simulink model "Qtank"  (R2016b)
settings: Solver=ode45  StartTime=0.0  StopTime=200.0  FixedStep=0.1  RelTol=1e-3
values from neighbouring files (symbols this model uses):
  a1 = 0.071    [datos.m]
  A1 = 28    [datos.m]
  A2 = 32    [datos.m]
  a2 = 0.057    [datos.m]
  A3 = 28    [datos.m]
  a3 = 0.071    [datos.m]
  A4 = 32    [datos.m]
  a4 = 0.057    [datos.m]
  g = 981    [datos.m]
  h1_0 = 40    [datos.m]
  h2_0 = 40    [datos.m]
  h3_0 = 40    [datos.m]
  h4_0 = 40    [datos.m]
  k1 = 3.33    [datos.m]
  k2 = 3.33    [datos.m]
  y1 = 0.7    [datos.m]
  y2 = 0.6    [datos.m]
libraries: simulink x2
settings Model: Creator=mathiaslambert  LastModifiedBy=mathiaslambert

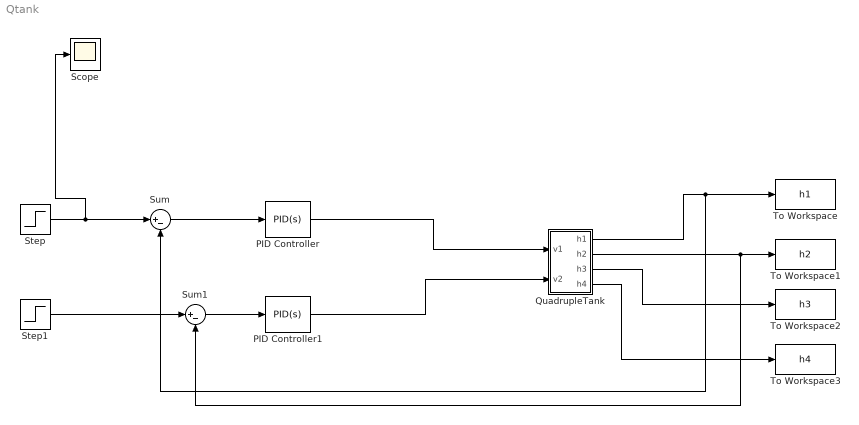
== system Qtank ==
  PID Controller : simulink/Continuous/PID Controller  Controller=PID  TimeDomain=Continuous-time  SampleTime=-1  IntegratorMethod=Forward Euler  FilterMethod=Forward Euler  Form=Parallel  UseFilter=on  ControllerParametersSource=internal  P=0.556896851749042  I=0.0082561633010969  D=-3.05414706908049  N=0.18234120333855  InitialConditionSource=internal  InitialConditionForIntegrator=0  InitialConditionForFilter=0  ExternalReset=none  LimitOutput=on  UpperSaturationLimit=5  LowerSaturationLimit=-5  LinearizeAsGain=on  AntiWindupMode=none  Kb=0.01  TrackingMode=off  Kt=1  PParamMin=[]  PParamMax=[]  IParamMin=[]  IParamMax=[]  DParamMin=[]  DParamMax=[]  NParamMin=[]  NParamMax=[]  KbParamMin=[]  KbParamMax=[]  KtParamMin=[]  KtParamMax=[]  POutMin=[]  POutMax=[]  IOutMin=[]  IOutMax=[]  DOutMin=[]  DOutMax=[]  NOutMin=[]  NOutMax=[]  KbOutMin=[]  KbOutMax=[]  KtOutMin=[]  KtOutMax=[]  IntegratorOutMin=[]  IntegratorOutMax=[]  FilterOutMin=[]  FilterOutMax=[]  SumOutMin=[]  SumOutMax=[]  SumI1OutMin=[]  SumI1OutMax=[]  SumI2OutMin=[]  SumI2OutMax=[]  SumI3OutMin=[]  SumI3OutMax=[]  SumDOutMin=[]  SumDOutMax=[]  SaturationOutMin=[]  SaturationOutMax=[]  IntegratorContinuousStateAttributes=''  IntegratorStateMustResolveToSignalObject=off  IntegratorRTWStateStorageClass=Auto  FilterContinuousStateAttributes=''  FilterStateMustResolveToSignalObject=off  FilterRTWStateStorageClass=Auto  DifferentiatorICPrevScaledInput=0  DifferentiatorOutMin=[]  DifferentiatorOutMax=[]
  PID Controller1 : simulink/Continuous/PID Controller  Controller=PID  TimeDomain=Continuous-time  SampleTime=-1  IntegratorMethod=Forward Euler  FilterMethod=Forward Euler  Form=Parallel  UseFilter=on  ControllerParametersSource=internal  P=1.02825937558598  I=0.0188425600987608  D=-0.134962487418389  N=7.61885317361069  InitialConditionSource=internal  InitialConditionForIntegrator=0  InitialConditionForFilter=0  ExternalReset=none  LimitOutput=on  UpperSaturationLimit=5  LowerSaturationLimit=-5  LinearizeAsGain=on  AntiWindupMode=none  Kb=0.01  TrackingMode=off  Kt=1  PParamMin=[]  PParamMax=[]  IParamMin=[]  IParamMax=[]  DParamMin=[]  DParamMax=[]  NParamMin=[]  NParamMax=[]  KbParamMin=[]  KbParamMax=[]  KtParamMin=[]  KtParamMax=[]  POutMin=[]  POutMax=[]  IOutMin=[]  IOutMax=[]  DOutMin=[]  DOutMax=[]  NOutMin=[]  NOutMax=[]  KbOutMin=[]  KbOutMax=[]  KtOutMin=[]  KtOutMax=[]  IntegratorOutMin=[]  IntegratorOutMax=[]  FilterOutMin=[]  FilterOutMax=[]  SumOutMin=[]  SumOutMax=[]  SumI1OutMin=[]  SumI1OutMax=[]  SumI2OutMin=[]  SumI2OutMax=[]  SumI3OutMin=[]  SumI3OutMax=[]  SumDOutMin=[]  SumDOutMax=[]  SaturationOutMin=[]  SaturationOutMax=[]  IntegratorContinuousStateAttributes=''  IntegratorStateMustResolveToSignalObject=off  IntegratorRTWStateStorageClass=Auto  FilterContinuousStateAttributes=''  FilterStateMustResolveToSignalObject=off  FilterRTWStateStorageClass=Auto  DifferentiatorICPrevScaledInput=0  DifferentiatorOutMin=[]  DifferentiatorOutMax=[]
  QuadrupleTank : Subsystem
  Scope : Scope
  Step : Step  Time=100  Before=40  After=45  SampleTime=0
  Step1 : Step  Time=100  Before=40  After=45  SampleTime=0
  Sum : Sum  Inputs=|+-
  Sum1 : Sum  Inputs=|+-
  To Workspace : ToWorkspace  VariableName=h1  SaveFormat=Timeseries  SampleTime=-1
  To Workspace1 : ToWorkspace  VariableName=h2  SaveFormat=Timeseries  SampleTime=-1
  To Workspace2 : ToWorkspace  VariableName=h3  SaveFormat=Timeseries  SampleTime=-1
  To Workspace3 : ToWorkspace  VariableName=h4  SaveFormat=Timeseries  SampleTime=-1
  wires:
  QuadrupleTank/1(h1) -> Sum/2, To Workspace/1
  QuadrupleTank/2(h2) -> Sum1/2, To Workspace1/1
  QuadrupleTank/3(h3) -> To Workspace2/1
  QuadrupleTank/4(h4) -> To Workspace3/1
  Step1/1 -> Sum1/1
  Step/1 -> Scope/1, Sum/1
  Sum1/1 -> PID Controller1/1
  Sum/1 -> PID Controller/1
  PID Controller/1 -> QuadrupleTank/1(v1)
  PID Controller1/1 -> QuadrupleTank/2(v2)

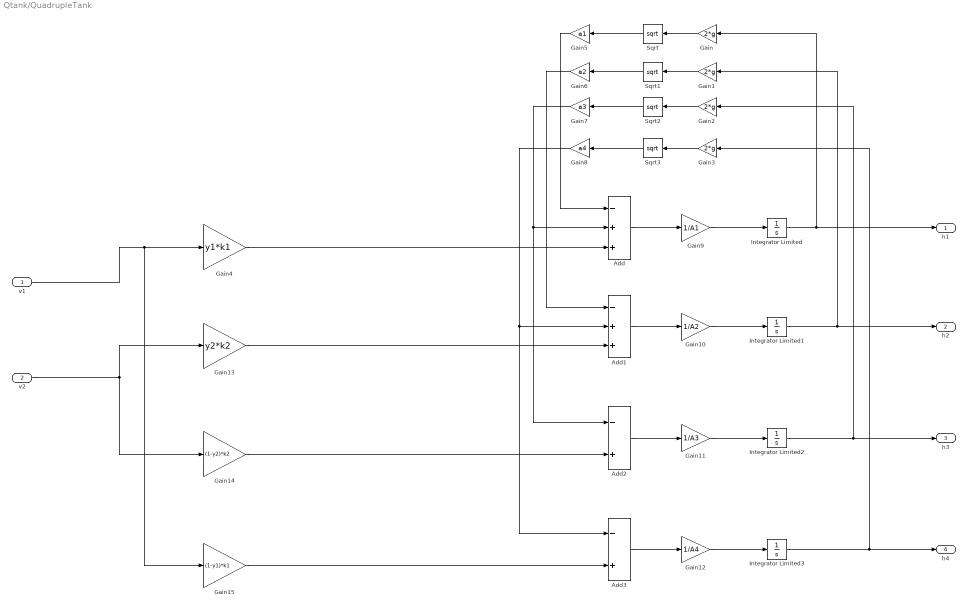
== system Qtank/QuadrupleTank ==
  v1 : Inport
  v2 : Inport  Port=2
  Add : Sum  Inputs=-++
  Add1 : Sum  Inputs=-++
  Add2 : Sum  Inputs=-+
  Add3 : Sum  Inputs=-+
  Gain{,1..3} (4 alike) : Gain  Gain=2*g
  Gain10 : Gain  Gain=1/A2
  Gain11 : Gain  Gain=1/A3
  Gain12 : Gain  Gain=1/A4
  Gain13 : Gain  Gain=y2*k2
  Gain14 : Gain  Gain=(1-y2)*k2
  Gain15 : Gain  Gain=(1-y1)*k1
  Gain4 : Gain  Gain=y1*k1
  Gain5 : Gain  Gain=a1
  Gain6 : Gain  Gain=a2
  Gain7 : Gain  Gain=a3
  Gain8 : Gain  Gain=a4
  Gain9 : Gain  Gain=1/A1
  Integrator Limited : Integrator  InitialCondition=h1_0  LimitOutput=on  UpperSaturationLimit=50  LowerSaturationLimit=0.01
  Integrator Limited1 : Integrator  InitialCondition=h2_0  LimitOutput=on  UpperSaturationLimit=50  LowerSaturationLimit=0.01
  Integrator Limited2 : Integrator  InitialCondition=h3_0  LimitOutput=on  UpperSaturationLimit=50  LowerSaturationLimit=0.01
  Integrator Limited3 : Integrator  InitialCondition=h4_0  LimitOutput=on  UpperSaturationLimit=50  LowerSaturationLimit=0.01
  Sqrt{,1..3} (4 alike) : Sqrt  SaturateOnIntegerOverflow=on
  h1 : Outport
  h2 : Outport  Port=2
  h3 : Outport  Port=3
  h4 : Outport  Port=4
  wires:
  Sqrt1/1 -> Gain6/1
  Sqrt3/1 -> Gain8/1
  Gain2/1 -> Sqrt2/1
  Gain/1 -> Sqrt/1
  Gain1/1 -> Sqrt1/1
  Gain7/1 -> Add/2, Add2/1
  Gain14/1 -> Add2/2
  Gain6/1 -> Add1/1
  Sqrt2/1 -> Gain7/1
  Sqrt/1 -> Gain5/1
  v2/1 -> Gain14/1, Gain13/1
  Integrator Limited3/1 -> h4/1, Gain3/1
  Integrator Limited/1 -> h1/1, Gain/1
  Gain10/1 -> Integrator Limited1/1
  v1/1 -> Gain15/1, Gain4/1
  Add2/1 -> Gain11/1
  Integrator Limited2/1 -> h3/1, Gain2/1
  Gain15/1 -> Add3/2
  Gain12/1 -> Integrator Limited3/1
  Integrator Limited1/1 -> h2/1, Gain1/1
  Gain4/1 -> Add/3
  Gain5/1 -> Add/1
  Gain11/1 -> Integrator Limited2/1
  Gain9/1 -> Integrator Limited/1
  Gain8/1 -> Add1/2, Add3/1
  Add1/1 -> Gain10/1
  Gain13/1 -> Add1/3
  Add/1 -> Gain9/1
  Add3/1 -> Gain12/1
  Gain3/1 -> Sqrt3/1
